simulink model "verify_sfun_storage_heatexchanger_mdl"  (Simulink 8.2)
settings: Solver=VariableStepDiscrete  StartTime=0.0  StopTime=1  MaxStep=1  RelTol=1e-3
values from neighbouring files (symbols this model uses):
  uam = 0.226    [verify_sfun_storage_heatexchanger2.m]
  uat = 0.550    (= 0.55)    [verify_sfun_storage_heatexchanger2.m]
undefined symbols (not defined in the file or in its folder): ua0
libraries: carnot x5
settings Model: Creator=drhf  LastModifiedBy=drhf

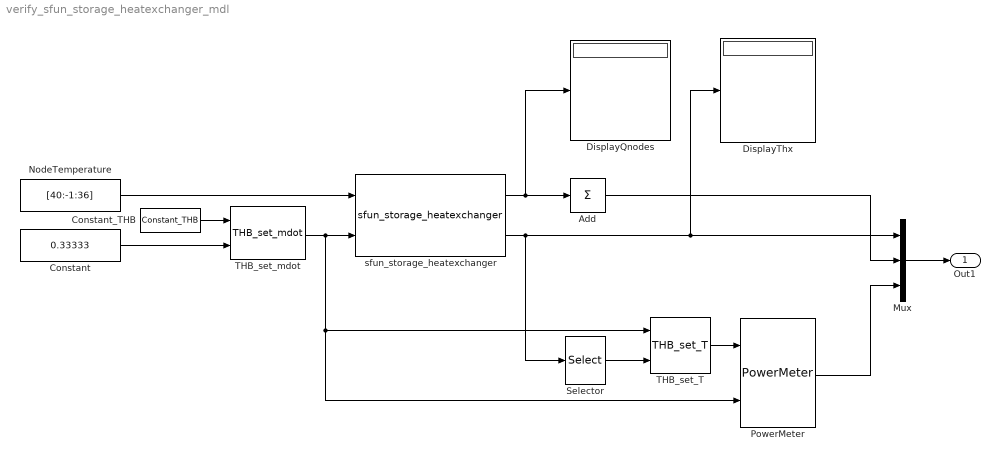
== system verify_sfun_storage_heatexchanger_mdl ==
  Add : Sum  Inputs=1
  Constant : Constant  Value=0.33333
  Constant_THB : carnot/Source/Simple/Constant_THB  t=40  mdot=1/3600  p=1e5  mID=No Pressure Drop  fluid=Water  mix=0  dia=0.02  hgt=0
  DisplayQnodes : Display
  DisplayThx : Display
  Mux : Mux  Inputs=3
  NodeTemperature : Constant  Value=[40:-1:36]
  PowerMeter : carnot/Control/PowerMeter
  Selector : Selector  InputPortWidth=5  IndexOptions=Index vector (dialog)  Indices=5  OutputSizes=1
  THB_set_T : carnot/Source/Simple/THB_set_T
  THB_set_mdot : carnot/Source/Simple/THB_set_mdot
  sfun_storage_heatexchanger : carnot/Basic/Thermal_Models/sfun_storage_heatexchanger  idn=heat transfer from data fit  nodes=5  inlet=1  outlet=5  pp=[100, 0, 0, 0,0,0,0] % [ua0, uam, uat, 0,0,0,0]
  Out1 : Outport
  wires:
  NodeTemperature/1 -> sfun_storage_heatexchanger/1
  sfun_storage_heatexchanger/1 -> DisplayQnodes/1, Add/1
  sfun_storage_heatexchanger/2 -> DisplayThx/1, Mux/1, Selector/1
  Constant_THB/1 -> THB_set_mdot/1
  THB_set_mdot/1 -> sfun_storage_heatexchanger/2, THB_set_T/1, PowerMeter/2
  Constant/1 -> THB_set_mdot/2
  Mux/1 -> Out1/1
  THB_set_T/1 -> PowerMeter/1
  PowerMeter/1 -> Mux/3
  Add/1 -> Mux/2
  Selector/1 -> THB_set_T/2
